simulink model "ModeSwitch"  (R2012b)
settings: configuration reference "configSetObj_autopilot" (kept outside this file)
settings Model: Creator=ssauvage  LastModifiedBy=ssauvage

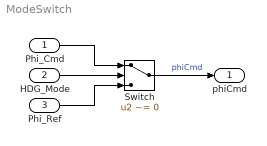
== system ModeSwitch ==
  Phi_Cmd : Inport  RequirementInfo={} %GIDa_d69514ae_5c9f_4aaf_9a57_91098752af65  OutDataTypeStr=double
  HDG_Mode : Inport  RequirementInfo={} %GIDa_10f04168_2496_438b_8d5f_b2518e76c840  Port=2  OutDataTypeStr=boolean
  Phi_Ref : Inport  RequirementInfo={} %GIDa_7b82ab37_d13a_4e76_b9de_794e33a8e441  Port=3  OutDataTypeStr=double
  Switch : Switch  RequirementInfo={} %GIDa_177a44a5_ab42_4901_a2bd_e87cb50f416d  Criteria=u2 ~= 0
  phiCmd : Outport  RequirementInfo={} %GIDa_e45e3dfe_1bf7_4b35_9371_03d183d0fb0a  OutDataTypeStr=double
  wires:
  Phi_Cmd/1 -> Switch/1
  HDG_Mode/1 -> Switch/2
  Switch/1 -> phiCmd/1  "phiCmd"
  Phi_Ref/1 -> Switch/3
